simulink model "inverse_GSFR_Individual_Vars"  (R2019b)
settings: Solver=VariableStepAuto  StartTime=0.0  StopTime=20  MaxStep=0.01  RelTol=1e-3
values from neighbouring files (symbols this model uses):
  a1 = (D*R+K)*2*c*wn    [dpt_from_dft_H.m]
  b1 = wn^2    [dpt_from_dft_H.m]
  c = (((2*H*R)+(((D*R)+(K*Fh))*Tr))/(2*(D*R+K)))*wn    [dpt_from_dft_H.m]
  c1 = (wn^2)*R*Tr    [dpt_from_dft_H.m]
  D = 1.0    (= 1)    [dpt_from_dft_H.m]
  d1 = (wn^2)*R    [dpt_from_dft_H.m]
  K = 0.95    [dpt_from_dft_H.m]
  R = 0.05    [dpt_from_dft_H.m]
  Tr = 8.0    (= 8)    [dpt_from_dft_H.m]
  wn = sqrt((D*R+K)/(2*H*R*Tr))    [dpt_from_dft_H.m]
  x1 = D*R+K    (= 1)    [dpt_from_dft_H.m]
settings Model: Creator=ruiva  LastModifiedBy=ruiva

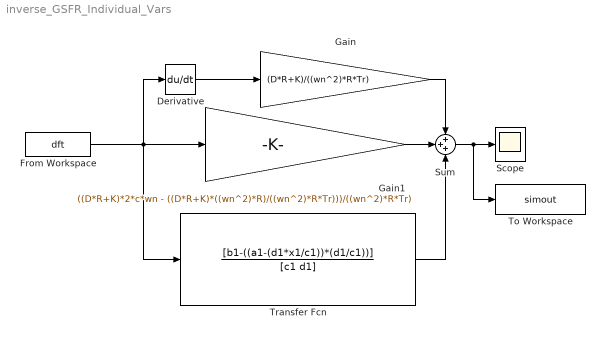
== system inverse_GSFR_Individual_Vars ==
  Derivative : Derivative
  From Workspace : FromWorkspace  VariableName=dft  SampleTime=0
  Gain : Gain  Gain=(D*R+K)/((wn^2)*R*Tr)
  Gain1 : Gain  Gain=((D*R+K)*2*c*wn - ((D*R+K)*((wn^2)*R)/((wn^2)*R*Tr)))/((wn^2)*R*Tr)
  Scope : Scope
  Sum : Sum  Inputs=+++
  To Workspace : ToWorkspace  VariableName=simout  SaveFormat=Timeseries  SampleTime=-1
  Transfer Fcn : TransferFcn  Numerator=[b1-((a1-(d1*x1/c1))*(d1/c1))]  Denominator=[c1 d1]
  wires:
  Derivative/1 -> Gain/1
  From Workspace/1 -> Transfer Fcn/1, Gain1/1, Derivative/1
  Transfer Fcn/1 -> Sum/3
  Gain1/1 -> Sum/2
  Gain/1 -> Sum/1
  Sum/1 -> To Workspace/1, Scope/1
